simulink model "automotive_console"  (R2020b)
settings: Solver=VariableStepAuto  StartTime=0.0  StopTime=10.0  RelTol=1e-3
settings Model: Creator=Milind  LastModifiedBy=Training

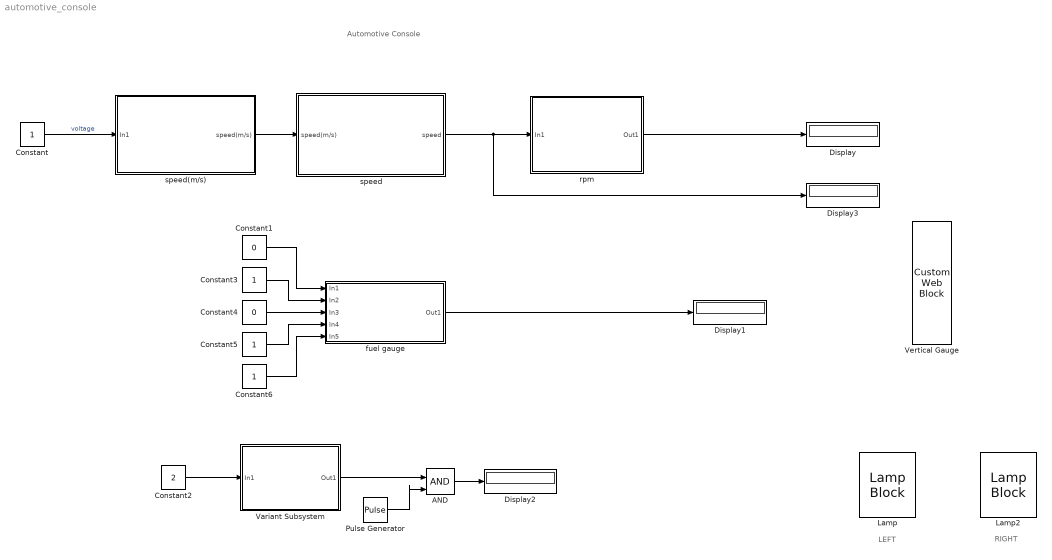
== system automotive_console ==
  note: Automotive Console
  note: RIGHT
  note: LEFT
  AND : Logic  IconShape=distinctive  AllPortsSameDT=off  OutDataTypeStr=boolean
  Constant{,3,5..6} (4 alike) : Constant
  Constant1 : Constant  Value=0
  Constant2 : Constant  Value=2
  Constant4 : Constant  Value=0
  Display{,1..3} (4 alike) : Display
  Lamp : LampBlock
  Lamp2 : LampBlock
  Pulse Generator : DiscretePulseGenerator  PulseType=Time based  Period=10  PulseWidth=50
  Variant Subsystem : Subsystem  Variant=on
  Vertical Gauge : CustomWebBlock  ShowInitialText=on  Configuration="{\"components\":[{\"name\":\"LinearScaleComponent\",\"settings\":{\"bounds\":{\"max\":5,\"min\":0,\"tickInterval\":\"auto\"},\"internalTickHeightScaleFactor\":0.5,\"labelColor\":[250,245,199],\"labelFont\":{\"font\":\"Arial\",\"fontSize\":12},\"labelTransparency\":1,\"needleImage\":{\"size\":[21,75],\"src\":\"data:image\\/svg+xml;base64,PHN2ZyB4bWxucz0iaHR0cDovL3d3dy53My5vcmcvMjAwMC9zdmciIHhtbG5zOnhsaW5rPSJodHRwOi8vd3d3LnczLm9yZy8xOTk5L3hsaW5rIiB2aWV3Qm94PSIwIDAgMjEgNzUiPjxkZWZzPjxzdHlsZT4uY2xzLTF7ZmlsbDpub25lO30uY2xzLTJ7aXNvbGF0aW9uOmlzb2xhdGU7fS5jbHMtM3tjbGlwLXBhdGg6dXJsKCNjbGlwLXBhdGgpO30uY2xzLTR7b3BhY2l0eTowLjM7bWl4LWJsZW5kLW1vZGU6bXVsdGlwbHk7fS5jbHMtNXtmaWxsOiNlYjI2Mjk7fTwvc3R5bGU+PGNsaXBQYXRoIGlkPSJjbGlwLXBhdGgiIHRyYW5zZm9y ...(+1928 chars)\",\"srcOrientation\":\"horizontal\"},\"needleOffset\":[-0.01094391244870041,0],\"needleSize\":{\"height\":0.11960078534031414,\"width\":0.7589285714285714},\"position\":[0.015887605042016806,0.06986607142857143,0.8,0.9641544117647058],\"scaleColors\":[],\"scaleColorsSize\":0.2,\"showLabels\":1,\"showMinorTicks\":0,\"showSpanLine\":1,\"showTicks\":1,\"tickColor\":[250,245,200],\"tickTransparency\":1,\"valueBarColor\":[23,89,176],\"valueBarOffset\":0,\"valueBarSize\":0.23,\"valueBarTransparency\":1}},{\"name\":\"BackgroundImageComponent\",\"settings\":{\"image\":{\"size\":[101,380],\"src\":\"data:image\\/svg+xml;base64,PHN2ZyB4bWxucz0iaHR0cDovL3d3dy53My5vcmcvMjAwMC9zdmciIHZpZXdCb3g9IjAgMCAxMDEgMzgwIj48ZGVmcz48c3R5bGU+LmNscy0xe2ZpbGw6IzAwMmI0Mjt9LmNscy0ye2ZpbGw6IzQyNzA4Mjt9LmNscy0ze2ZpbGw6IzdjYTBiMjt9PC9zdHlsZT48L2RlZnM+PHRpdGxlPnZlcnRpY2FsX2dhdWdlX2JhY2tncm91bmRfMTwvdGl0bGU+PGcgaWQ9IkxheWVyXzIiIGRhdGEtbmFtZT0iTGF5ZXIgMiI+PGcgaWQ9IkxheWVyXzEtMiIgZGF0YS1uYW1lPSJMYXllciAxIj48cmVjdCBjbGFzcz0iY2xzLTEiIHg9IjExIiB5PSIxMSIgd2lkdGg9Ijc5IiBoZWlnaHQ9IjM1OCIvPjxwYXRoIGNsYXNzPSJjbHMtMiIgZD0iTTkzLDhIOFYzNzJIOTNaTTExLDM2OVYxMUg5MFYzNjlaIi8+PHBhdGggY2xhc3M9ImNscy0zIiBkPSJNMTAxLDBIMFYzODBIMTAxWk04LDM3MlY4SDkzVjM3MloiLz48L2c+PC9nPjwvc3ZnPg==\",\"srcOrientation\":\"vertical\"},\"position\":[0,0,1,1],\"scaleMode\":\"0\"}},{\"name\":\"ForegroundImageComponent\",\"settings\":{\"image\":{\"size\":[0,0],\"src\":\"default\",\"srcOrientation\":[]},\"isForeground\":1,\"position\":[0,0,1,1],\"scaleMode\":\"0\"}}],\"settings\":{\"BindingType\":\"signal\",\"aspectRatio\":0.2648221343873518,\"fixedAspectRatio\":\"on\",\"orientation\":\"vertical\"},\"type\":\"LinearGauge\"}"
  fuel gauge : Subsystem
  rpm : Subsystem  Variant=on
  speed : Subsystem  Variant=on  AllowZeroVariantControls=on
  speed(m/s) : Subsystem
  wires:
  fuel gauge/1(Out1) -> Display1/1
  Constant1/1 -> fuel gauge/1(In1)
  Constant3/1 -> fuel gauge/2(In2)
  Constant4/1 -> fuel gauge/3(In3)
  Constant5/1 -> fuel gauge/4(In4)
  Constant6/1 -> fuel gauge/5(In5)
  rpm/1(Out1) -> Display/1
  speed/1(speed) -> Display3/1, rpm/1(In1)
  speed(m/s)/1(speed(m/s)) -> speed/1(speed(m/s))
  Constant/1 -> speed(m/s)/1(In1)  "voltage"
  AND/1 -> Display2/1
  Pulse Generator/1 -> AND/2
  Constant2/1 -> Variant Subsystem/1(In1)
  Variant Subsystem/1(Out1) -> AND/1

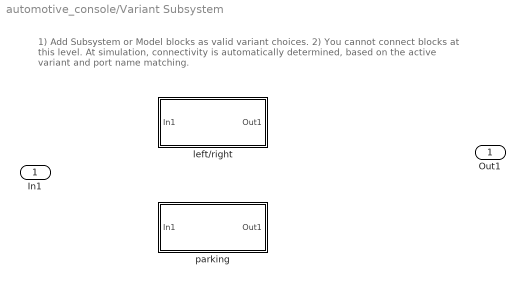
== system automotive_console/Variant Subsystem ==
  note: 1) Add Subsystem or Model blocks as valid variant choices.
      | 2) You cannot connect blocks at this level. At simulation, connectivity is automatically
      | determined, based on the active variant and port name matching.
  In1 : Inport
  left/right : Subsystem  VariantControl=ind==0
  parking : Subsystem  VariantControl=ind==1
  Out1 : Outport

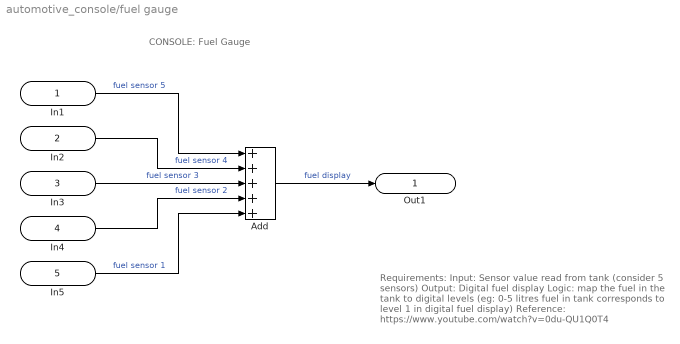
== system automotive_console/fuel gauge ==
  note: CONSOLE: Fuel Gauge
  note: Requirements:
      | Input: Sensor value read from tank (consider 5 sensors)
      | Output: Digital fuel display
      | Logic: map the fuel in the tank to digital levels (eg: 0-5 litres fuel in tank corresponds to level 1 in digital fuel display) Reference: https://www.youtube.com/watch?v=0du-QU1Q0T4
  In1 : Inport
  In2 : Inport  Port=2
  In3 : Inport  Port=3
  In4 : Inport  Port=4
  In5 : Inport  Port=5
  Add : Sum  Inputs=+++++
  Out1 : Outport
  wires:
  Add/1 -> Out1/1  "fuel display"
  In1/1 -> Add/1  "fuel sensor 5"
  In2/1 -> Add/2  "fuel sensor 4"
  In3/1 -> Add/3  "fuel sensor 3"
  In4/1 -> Add/4  "fuel sensor 2"
  In5/1 -> Add/5  "fuel sensor 1"

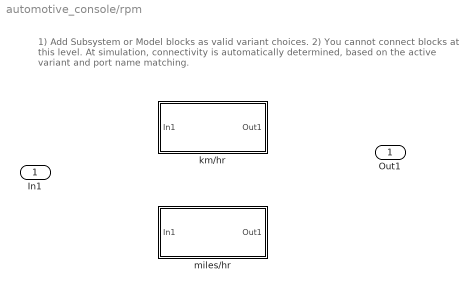
== system automotive_console/rpm ==
  note: 1) Add Subsystem or Model blocks as valid variant choices.
      | 2) You cannot connect blocks at this level. At simulation, connectivity is automatically
      | determined, based on the active variant and port name matching.
  In1 : Inport
  km/hr : Subsystem  VariantControl=control==0
  miles/hr : Subsystem  VariantControl=control==1
  Out1 : Outport

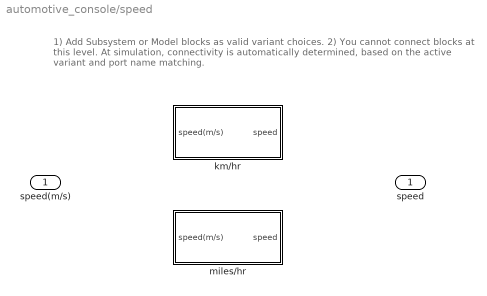
== system automotive_console/speed ==
  note: 1) Add Subsystem or Model blocks as valid variant choices.
      | 2) You cannot connect blocks at this level. At simulation, connectivity is automatically
      | determined, based on the active variant and port name matching.
  speed(m/s) : Inport
  km/hr : Subsystem  VariantControl=control==0
  miles/hr : Subsystem  VariantControl=control==1
  speed : Outport

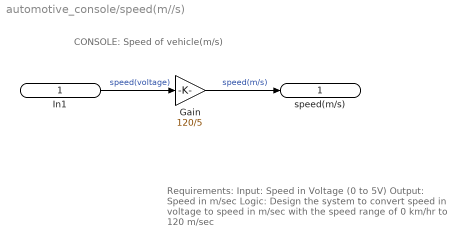
== system automotive_console/speed(m//s) ==
  note: CONSOLE: Speed of vehicle(m/s)
  note: Requirements:
      | Input: Speed in Voltage (0 to 5V)
      | Output: Speed in m/sec
      | Logic: Design the system to convert speed in voltage to
      | speed in m/sec with the speed range of 0 km/hr to 120 m/sec
  In1 : Inport
  Gain : Gain  Gain=120/5
  speed(m/s) : Outport
  wires:
  In1/1 -> Gain/1  "speed(voltage)"
  Gain/1 -> speed(m/s)/1  "speed(m/s)"

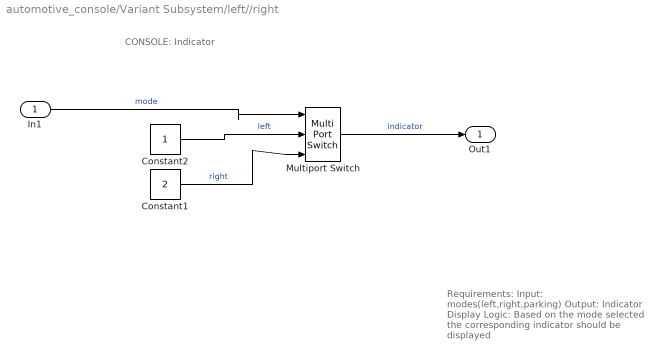
== system automotive_console/Variant Subsystem/left//right ==
  note: Requirements:
      | Input: modes(left,right,parking)
      | Output: Indicator Display
      | Logic: Based on the mode selected the corresponding indicator should be displayed
  note: CONSOLE: Indicator
  In1 : Inport
  Constant1 : Constant  Value=2
  Constant2 : Constant
  Multiport Switch : MultiPortSwitch  Inputs=2
  Out1 : Outport
  wires:
  In1/1 -> Multiport Switch/1  "mode"
  Constant1/1 -> Multiport Switch/3  "right"
  Constant2/1 -> Multiport Switch/2  "left"
  Multiport Switch/1 -> Out1/1  "indicator"

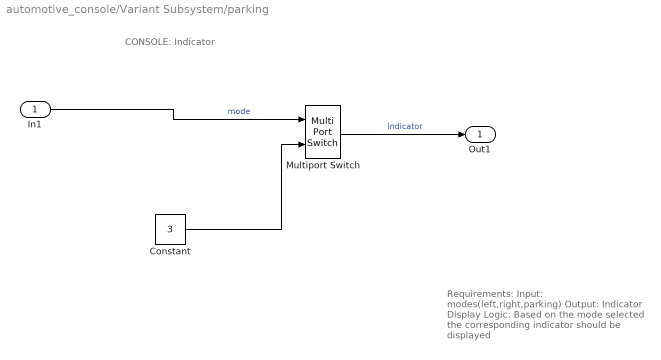
== system automotive_console/Variant Subsystem/parking ==
  note: Requirements:
      | Input: modes(left,right,parking)
      | Output: Indicator Display
      | Logic: Based on the mode selected the corresponding indicator should be displayed
  note: CONSOLE: Indicator
  In1 : Inport
  Constant : Constant  Value=3
  Multiport Switch : MultiPortSwitch  Inputs=1
  Out1 : Outport
  wires:
  Constant/1 -> Multiport Switch/2
  In1/1 -> Multiport Switch/1  "mode"
  Multiport Switch/1 -> Out1/1  "indicator"

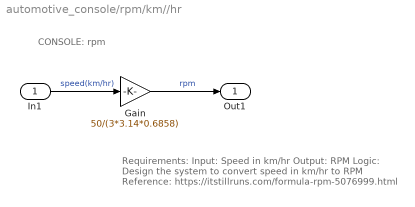
== system automotive_console/rpm/km//hr ==
  note: Requirements:
      | Input: Speed in km/hr
      | Output: RPM
      | Logic: Design the system to convert speed in km/hr to RPM Reference: https://itstillruns.com/formula-rpm-5076999.html
  note: CONSOLE: rpm
  In1 : Inport
  Gain : Gain  Gain=50/(3*3.14*0.6858)
  Out1 : Outport
  wires:
  Gain/1 -> Out1/1  "rpm"
  In1/1 -> Gain/1  "speed(km/hr)"

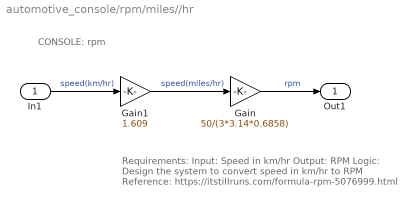
== system automotive_console/rpm/miles//hr ==
  note: Requirements:
      | Input: Speed in km/hr
      | Output: RPM
      | Logic: Design the system to convert speed in km/hr to RPM Reference: https://itstillruns.com/formula-rpm-5076999.html
  note: CONSOLE: rpm
  In1 : Inport
  Gain : Gain  Gain=50/(3*3.14*0.6858)
  Gain1 : Gain  Gain=1.609
  Out1 : Outport
  wires:
  Gain/1 -> Out1/1  "rpm"
  In1/1 -> Gain1/1  "speed(km/hr)"
  Gain1/1 -> Gain/1  "speed(miles/hr)"

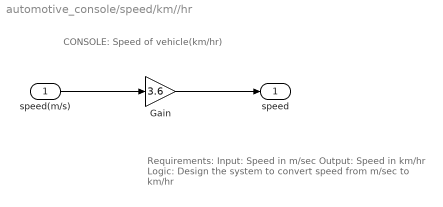
== system automotive_console/speed/km//hr ==
  note: Requirements:
      | Input: Speed in m/sec
      | Output: Speed in km/hr
      | Logic: Design the system to convert speed from m/sec to km/hr
  note: CONSOLE: Speed of vehicle(km/hr)
  speed(m/s) : Inport
  Gain : Gain  Gain=3.6
  speed : Outport
  wires:
  Gain/1 -> speed/1
  speed(m/s)/1 -> Gain/1

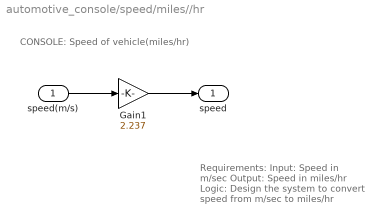
== system automotive_console/speed/miles//hr ==
  note: Requirements:
      | Input: Speed in m/sec
      | Output: Speed in miles/hr
      | Logic: Design the system to convert speed from m/sec to miles/hr
  note: CONSOLE: Speed of vehicle(miles/hr)
  speed(m/s) : Inport
  Gain1 : Gain  Gain=2.237
  speed : Outport
  wires:
  Gain1/1 -> speed/1
  speed(m/s)/1 -> Gain1/1
